simulink model "signal_converter"  (R2021a)
settings: Solver=VariableStepAuto  StartTime=0.0  StopTime=10.0  RelTol=1e-3
settings Model: Creator=beave  LastModifiedBy=thana
settings SolverCC: AlgebraicLoopSolver=TrustRegion
settings DebuggingCC: SFMachineParentedDataDiag=warning

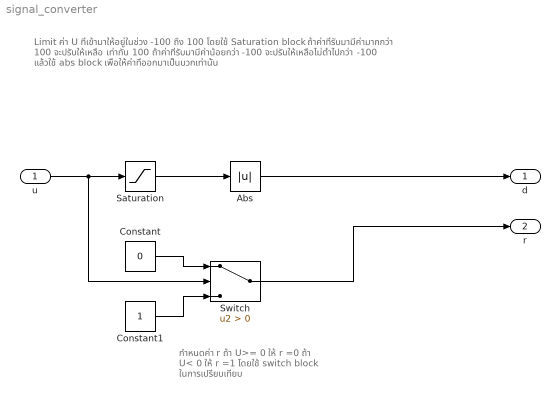
== system signal_converter ==
  note: Limit ค่า U ที่เข้ามาให้อยู่ในช่วง -100 ถึง 100
      | โดยใช้ Saturation block
      | ถ้าค่าที่รับมามีค่ามากกว่า 100 จะปรับให้เหลือ เท่ากับ 100
      | ถ้าค่าที่รับมามีค่าน้อยกว่า -100 จะปรับให้เหลือไม่ต่ำไปกว่า -100
      | แล้วใช้ abs block เพื่อให้ค่าที่ออกมาเป็นบวกเท่านั้น
  note: กำหนดค่า r
      | ถ้า U>= 0 ให้ r =0
      | ถ้า U< 0 ให้ r =1
      | โดยใช้ switch block
      | ในการเปรียบเทียบ
  u : Inport
  Abs : Abs
  Constant : Constant  Value=0
  Constant1 : Constant
  Saturation : Saturate  UpperLimit=100  LowerLimit=-100
  Switch : Switch  Criteria=u2 > Threshold
  d : Outport
  r : Outport  Port=2
  wires:
  u/1 -> Switch/2, Saturation/1
  Saturation/1 -> Abs/1
  Abs/1 -> d/1
  Constant/1 -> Switch/1
  Constant1/1 -> Switch/3
  Switch/1 -> r/1
